simulink model "modeloMovimiento"  (R2014a)
settings: Solver=ode45  StartTime=0.0  StopTime=10.0  RelTol=1e-6
settings Model: Creator=PedroBarquin  LastModifiedBy=PedroBarquin

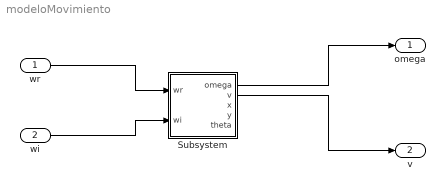
== system modeloMovimiento ==
  "wr " : Inport
  wi : Inport  Port=2
  Subsystem : Subsystem
  "omega " : Outport
  "v " : Outport  Port=2
  wires:
  "wr "/1 -> Subsystem/1("wr ")
  wi/1 -> Subsystem/2(wi)
  Subsystem/1("omega ") -> "omega "/1
  Subsystem/2("v ") -> "v "/1

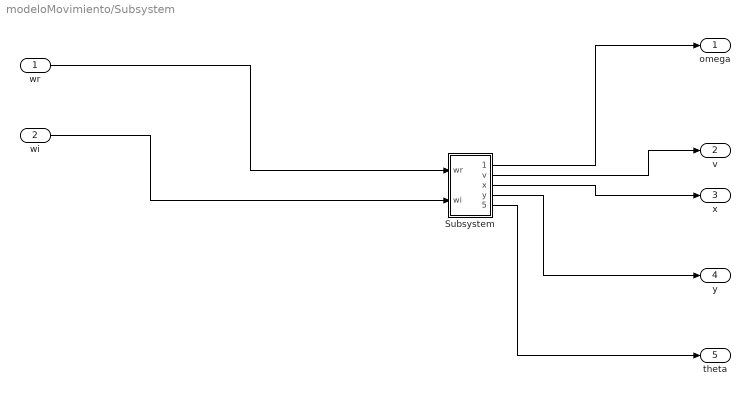
== system modeloMovimiento/Subsystem ==
  "wr " : Inport
  wi : Inport  Port=2
  Subsystem : Subsystem  mask{r=1, L=1, x_0=0, y_0=0, theta_0=0}
  "omega " : Outport
  "v " : Outport  Port=2
  "x " : Outport  Port=3
  "y " : Outport  Port=4
  "theta " : Outport  Port=5
  wires:
  "wr "/1 -> Subsystem/1("wr ")
  wi/1 -> Subsystem/2(wi)
  Subsystem/1("omega ") -> "omega "/1
  Subsystem/2("v ") -> "v "/1
  Subsystem/3("x ") -> "x "/1
  Subsystem/4("y ") -> "y "/1
  Subsystem/5("theta ") -> "theta "/1

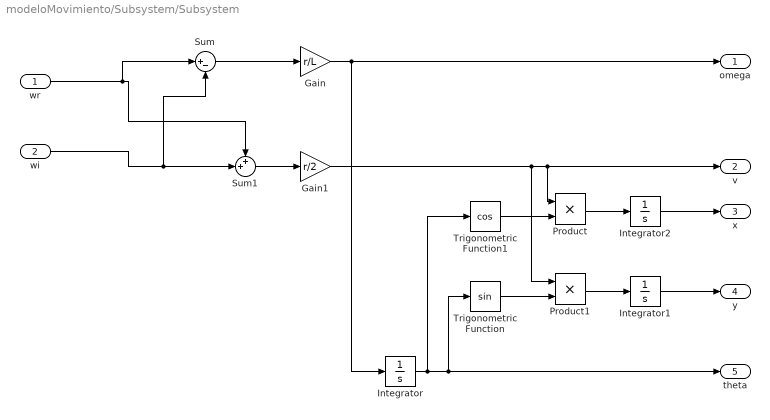
== system modeloMovimiento/Subsystem/Subsystem ==
  "wr " : Inport
  wi : Inport  Port=2
  Gain : Gain  Gain=r/L
  Gain1 : Gain  Gain=r/2
  Integrator : Integrator  InitialCondition=theta_0
  Integrator1 : Integrator  InitialCondition=y_0
  Integrator2 : Integrator  InitialCondition=x_0
  Product : Product
  Product1 : Product
  Sum : Sum  Inputs=|+-
  Sum1 : Sum  Inputs=++|
  Trigonometric Function : Trigonometry
  Trigonometric Function1 : Trigonometry  Operator=cos
  "omega " : Outport
  "v " : Outport  Port=2
  "x " : Outport  Port=3
  "y " : Outport  Port=4
  "theta " : Outport  Port=5
  wires:
  Gain/1 -> "omega "/1, Integrator/1
  Sum/1 -> Gain/1
  Gain1/1 -> Product1/1, "v "/1, Product/1
  Sum1/1 -> Gain1/1
  wi/1 -> Sum/2, Sum1/2
  "wr "/1 -> Sum/1, Sum1/1
  Trigonometric Function/1 -> Product1/2
  Trigonometric Function1/1 -> Product/2
  Product1/1 -> Integrator1/1
  Integrator/1 -> Trigonometric Function1/1, "theta "/1, Trigonometric Function/1
  Integrator1/1 -> "y "/1
  Product/1 -> Integrator2/1
  Integrator2/1 -> "x "/1
